simulink model "S250205simul_switch_2023a"  (R2024b)
settings: Solver=FixedStepDiscrete  StartTime=0  StopTime=60  FixedStep=0.01  RelTol=1e-3  AbsTol=1e-6
undefined symbols (not defined in the file or in its folder): a, b, c, d, f, g, switch_logic, VmcRgn_C_C, VmcRgn_J_C, VmcRgn_k_1to2_C, VmcRgn_k_2to3_C, VmcRgn_k_2to6_C, VmcRgn_k_3to4_C, VmcRgn_k_5to2_C, VmcRgn_k_6to2_C, VmcRgn_Kp_C, VmcRgn_L_C, VmcRgn_lf_C, VmcRgn_lr_C, VmcRgn_mass_C, VmcRgn_Mot2Whl_C, VmcRgn_PedDep_thrs_C, VmcRgn_phs2_k_C, VmcRgn_phs2_tq_C, VmcRgn_phs3_tq_C, VmcRgn_phs4_tq_C, VmcRgn_phs5_tq_C, VmcRgn_phs6_tq_C, VmcRgn_r_e_C, VmcRgn_R_whl_C, VmcRgn_SAS_thrs_C, VmcRgn_slip_max_C, VmcRgn_slip_max_gain_F_C, VmcRgn_slip_max_gain_R_C, VmcRgn_sup_tq_C, VmcRgn_t_pred_C, VmcRgn_target_w_acc_C, VmcRgn_tTs, VmcRgn_tTsinMs_C, VmcRgn_Yaw_thrs_C, yaw_flag
libraries: simulink x26, simulink_need_slupdate x1
(part 2 of 3)

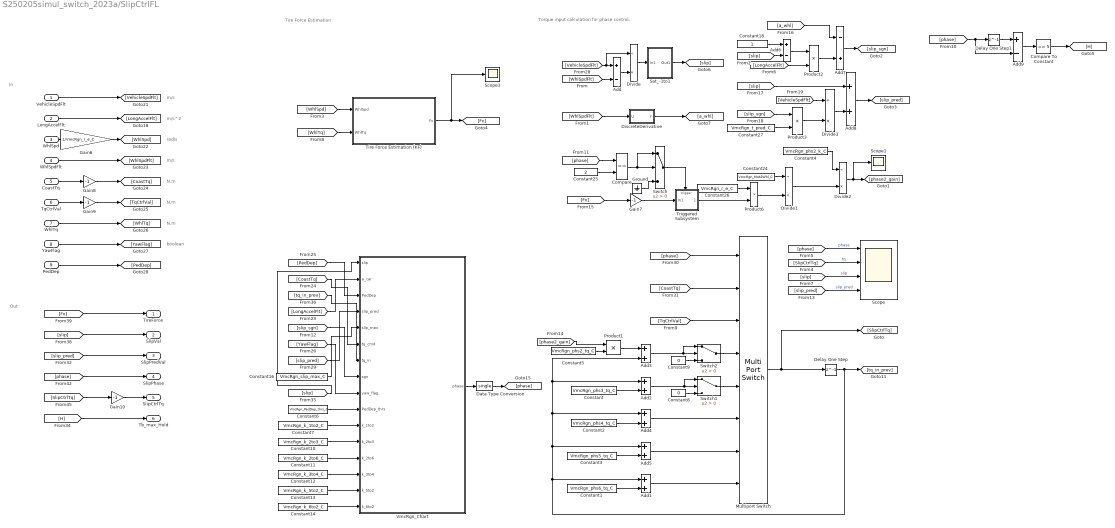
== system S250205simul_switch_2023a/SlipCtrlFL ==
  note: m/s
  note: N.m
  note: boolean
  note: N.m
  note: m/s
  note: Torque input calculation for phase control.
  note: Out
  note: N.m
  note: rad/s
  note: Tire Force Estimation
  note: m/s^2
  note: In
  VehicleSpdFlt : Inport
  LongAccelFlt : Inport  Port=2
  WhlSpd : Inport  Port=3
  WhlSpdFlt : Inport  Port=4
  CoastTq : Inport  Port=5
  TqCtrlVal : Inport  Port=6
  WhlTq : Inport  Port=7
  YawFlag : Inport  Port=8
  PedDep : Inport  Port=9
  Add : Sum  Inputs=+-
  Add{1..5,8} (6 alike) : Sum
  Add6 : Sum  Inputs=+-
  Add7 : Sum  Inputs=-+
  Add9 : Sum  Inputs=+-
  Compare : RelationalOperator  Operator===  OutDataTypeStr=boolean
  Compare To Constant : simulink/Logic and Bit Operations/Compare To Constant  relop===  const=5  OutDataTypeStr=boolean
  Constant : Constant  Value=VmcRgn_phs3_tq_C  OutDataTypeStr=single
  Constant1 : Constant  Value=VmcRgn_phs6_tq_C  OutDataTypeStr=single
  Constant10 : Constant  Value=VmcRgn_k_2to3_C  OutDataTypeStr=single
  Constant11 : Constant  Value=VmcRgn_k_2to6_C  OutDataTypeStr=single
  Constant12 : Constant  Value=VmcRgn_k_3to4_C  OutDataTypeStr=single
  Constant13 : Constant  Value=VmcRgn_k_5to2_C  OutDataTypeStr=single
  Constant14 : Constant  Value=VmcRgn_k_6to2_C  OutDataTypeStr=single
  Constant16 : Constant  Value=VmcRgn_slip_max_C  OutDataTypeStr=single
  Constant18 : Constant  OutDataTypeStr=single
  Constant2 : Constant  Value=VmcRgn_phs4_tq_C  OutDataTypeStr=single
  Constant24 : Constant  Value=VmcRgn_Mot2Whl_C  OutDataTypeStr=single
  Constant25 : Constant  Value=2  OutDataTypeStr=single
  Constant26 : Constant  Value=VmcRgn_r_e_C  OutDataTypeStr=single
  Constant27 : Constant  Value=VmcRgn_t_pred_C  OutDataTypeStr=single
  Constant3 : Constant  Value=VmcRgn_phs5_tq_C  OutDataTypeStr=single
  Constant4 : Constant  Value=VmcRgn_phs2_k_C  OutDataTypeStr=single
  Constant5 : Constant  Value=VmcRgn_phs2_tq_C  OutDataTypeStr=single
  Constant6 : Constant  Value=VmcRgn_PedDep_thrs_C  OutDataTypeStr=single
  Constant7 : Constant  Value=VmcRgn_k_1to2_C  OutDataTypeStr=single
  Constant8 : Constant  Value=0  OutDataTypeStr=single
  Constant9 : Constant  Value=0  OutDataTypeStr=single
  Data Type Conversion : DataTypeConversion  OutDataTypeStr=single  SaturateOnIntegerOverflow=off  RndMeth=Floor
  Delay One Step : Delay  DelayLength=1
  Delay One Step1 : Delay  DelayLength=1
  DiscreteDerivative : Subsystem  TreatAsAtomicUnit=on  RTWFileName=HmcLib_DebFlt  mask(Discrete Derivative with fixed sample time){Ts=VmcRgn_tTsinMs_C, out_type=single}
      mask prompts: Ts "Sampling Period [ms]"; out_type "Output DataType:"
      mask help:
      | Discrete-time derivative of the input.
      |
      | * Notes
      |   - Internal data type: Float32 (single)
      settings: AttributesFormatString=Sampling Period [ms]: %<Ts>\nOutType: %<out_type>  RTWSystemCode=Inline
  Divide : Product  Inputs=/*  OutDataTypeStr=single
  Divide1 : Product  Inputs=/*
  Divide2 : Product  Inputs=/*
  Divide3 : Product  Inputs=/*
  Gain{7..10} (4 alike) : Gain  Gain=-1
  Gain6 : Gain  Gain=1/VmcRgn_r_e_C
  Ground : Ground
  Multiport Switch : MultiPortSwitch  DataPortOrder=Zero-based contiguous  Inputs=7  zeroidx=on  OutDataTypeStr=single  SaturateOnIntegerOverflow=off  InputSameDT=off
  Product{1..3,6} (4 alike) : Product
  Sat_-1to1 : Subsystem
  Scope : Scope  NumInputPorts=4
  Scope1 : Scope
  Scope3 : Scope
  Switch : Switch  Criteria=u2 > Threshold  SaturateOnIntegerOverflow=off  InputSameDT=off
  Switch1 : Switch  Criteria=u2 > Threshold  SaturateOnIntegerOverflow=off  InputSameDT=off
  Switch2 : Switch  Criteria=u2 > Threshold  SaturateOnIntegerOverflow=off  InputSameDT=off
  Tire Force Estimation (KF) : Subsystem
  Triggered Subsystem : Subsystem  TreatAsAtomicUnit=on
  VmcRgn_Chart : Stateflow chart  TreatAsAtomicUnit=on
  TireForce : Outport
  SlipVal : Outport  Port=2
  SlipPredVal : Outport  Port=3
  SlipPhase : Outport  Port=4
  SlipCtrlTq : Outport  Port=5
  Tb_max_Hold : Outport  Port=6
  wires:
  [WhlSpd] -> Tire Force Estimation (KF)/1(WhlSpd)
  Data Type Conversion/1 -> [phase]
  Product3/1 -> Divide3/2
  Product2/1 -> Add7/2
  VmcRgn_Chart/1(phase) -> Data Type Conversion/1
  Divide3/1 -> Add8/2
  [slip] -> Add8/1
  [LongAccelFlt] -> Product2/2
  Switch2/1 -> Multiport Switch/4
  Add8/1 -> [slip_pred]
  Constant9/1 -> Switch2/3
  Delay One Step/1 -> [tq_in_prev], Add1/1, Add3/2, Add2/1, Add4/1, Add5/1
  [slip_sgn] -> Product3/1
  Constant26/1 -> Product6/1
  Triggered Subsystem/1(Out1) -> Product6/2
  Divide1/1 -> Divide2/2
  Constant4/1 -> Divide2/1
  Switch/1 -> Triggered Subsystem/Trigger
  Constant24/1 -> Divide1/1
  Product6/1 -> Divide1/2
  Ground/1 -> Switch/3
  [VehicleSpdFlt] -> Divide/1, Add/1
  Sat_-1to1/1(Out1) -> [slip]
  [WhlSpdFlt] -> DiscreteDerivative/1(U)
  [slip] -> Add6/2
  Constant1/1 -> Add1/2
  [slip_pred] -> Scope/4  "slip_pred"
  Add3/1 -> Switch2/1, Switch2/2
  [WhlTq] -> Tire Force Estimation (KF)/2(WhlTq)
  Add2/1 -> Switch1/1, Switch1/2
  [LongAccelFlt] -> VmcRgn_Chart/2(a_car)
  [SlipCtrlTq] -> Scope/2  "tq"
  [tq_in_prev] -> VmcRgn_Chart/7(tq_in)
  [WhlSpdFlt] -> Add/2
  [phase] -> Scope/1  "phase"
  Add6/1 -> Product2/1
  Gain8/1 -> [CoastTq]
  WhlSpd/1 -> Gain6/1
  YawFlag/1 -> [YawFlag]
  Multiport Switch/1 -> [SlipCtrlTq], Delay One Step/1
  CoastTq/1 -> Gain8/1
  Add4/1 -> Multiport Switch/6
  Constant3/1 -> Add5/2
  Divide/1 -> Sat_-1to1/1(In1)
  Constant27/1 -> Product3/2
  [phase] -> Compare/1
  Constant2/1 -> Add4/2
  Constant6/1 -> VmcRgn_Chart/10(PedDep_thrs)
  [phase2_gain] -> Product1/1
  [slip_sgn] -> VmcRgn_Chart/8(sgn)
  [slip] -> Scope/3  "slip"
  Constant/1 -> Add2/2
  Add5/1 -> Multiport Switch/7
  Constant14/1 -> VmcRgn_Chart/16(k_6to2)
  [YawFlag] -> VmcRgn_Chart/9(yaw_flag)
  Constant8/1 -> Switch1/3
  Constant10/1 -> VmcRgn_Chart/12(k_2to3)
  Constant7/1 -> VmcRgn_Chart/11(k_1to2)
  [CoastTq] -> VmcRgn_Chart/6(tq_cmd)
  [slip_pred] -> VmcRgn_Chart/4(slip_pred)
  Constant13/1 -> VmcRgn_Chart/15(k_5to2)
  Constant25/1 -> Compare/2
  Constant18/1 -> Add6/1
  [slip_pred] -> SlipPredVal/1
  Tire Force Estimation (KF)/1(Fx) -> Scope3/1, [Fx]
  Divide2/1 -> Scope1/1, [phase2_gain]
  Product1/1 -> Add3/1
  Gain6/1 -> [WhlSpd]
  Gain10/1 -> SlipCtrlTq/1
  Constant11/1 -> VmcRgn_Chart/13(k_2to6)
  LongAccelFlt/1 -> [LongAccelFlt]
  Compare/1 -> Switch/1, Switch/2
  [CoastTq] -> Multiport Switch/2
  Add7/1 -> [slip_sgn]
  Gain9/1 -> [TqCtrlVal]
  DiscreteDerivative/1(Y) -> [a_whl]
  [Fx] -> TireForce/1
  [slip] -> SlipVal/1
  [phase] -> SlipPhase/1
  WhlSpdFlt/1 -> [WhlSpdFlt]
  [SlipCtrlTq] -> Gain10/1
  WhlTq/1 -> [WhlTq]
  [slip] -> VmcRgn_Chart/1(slip)
  TqCtrlVal/1 -> Gain9/1
  [phase] -> Multiport Switch/1
  PedDep/1 -> [PedDep]
  Gain7/1 -> Triggered Subsystem/1(In1)
  [PedDep] -> VmcRgn_Chart/3(PedDep)
  [TqCtrlVal] -> Multiport Switch/3
  Constant12/1 -> VmcRgn_Chart/14(k_3to4)
  Switch1/1 -> Multiport Switch/5
  Add/1 -> Divide/2
  Add1/1 -> Multiport Switch/8
  [VehicleSpdFlt] -> Divide3/1
  VehicleSpdFlt/1 -> [VehicleSpdFlt]
  [Fx] -> Gain7/1
  Constant16/1 -> VmcRgn_Chart/5(slip_max)
  Constant5/1 -> Product1/2
  [a_whl] -> Add7/1
  [phase] -> Add9/2, Delay One Step1/1
  Compare To Constant/1 -> [H]
  Add9/1 -> Compare To Constant/1
  Delay One Step1/1 -> Add9/1
  [H] -> Tb_max_Hold/1

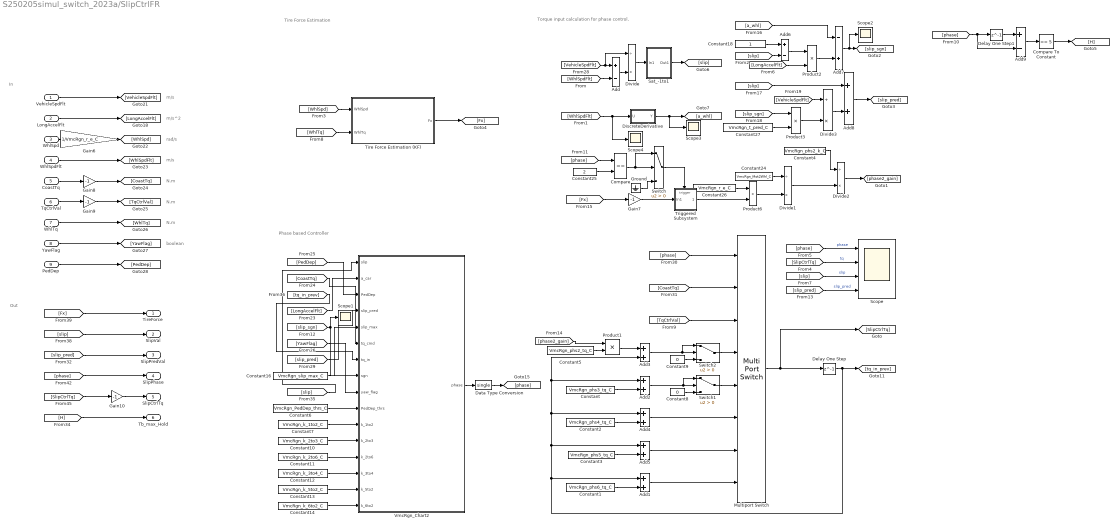
== system S250205simul_switch_2023a/SlipCtrlFR ==
  note: Phase based Controller
  note: m/s
  note: N.m
  note: boolean
  note: N.m
  note: m/s
  note: Torque input calculation for phase control.
  note: Out
  note: N.m
  note: rad/s
  note: Tire Force Estimation
  note: m/s^2
  note: In
  VehicleSpdFlt : Inport
  LongAccelFlt : Inport  Port=2
  WhlSpd : Inport  Port=3
  WhlSpdFlt : Inport  Port=4
  CoastTq : Inport  Port=5
  TqCtrlVal : Inport  Port=6
  WhlTq : Inport  Port=7
  YawFlag : Inport  Port=8
  PedDep : Inport  Port=9
  Add : Sum  Inputs=+-
  Add{1..5,8} (6 alike) : Sum
  Add6 : Sum  Inputs=+-
  Add7 : Sum  Inputs=-+
  Add9 : Sum  Inputs=+-
  Compare : RelationalOperator  Operator===  OutDataTypeStr=boolean
  Compare To Constant : simulink/Logic and Bit Operations/Compare To Constant  relop===  const=5  OutDataTypeStr=boolean
  Constant : Constant  Value=VmcRgn_phs3_tq_C  OutDataTypeStr=single
  Constant1 : Constant  Value=VmcRgn_phs6_tq_C  OutDataTypeStr=single
  Constant10 : Constant  Value=VmcRgn_k_2to3_C  OutDataTypeStr=single
  Constant11 : Constant  Value=VmcRgn_k_2to6_C  OutDataTypeStr=single
  Constant12 : Constant  Value=VmcRgn_k_3to4_C  OutDataTypeStr=single
  Constant13 : Constant  Value=VmcRgn_k_5to2_C  OutDataTypeStr=single
  Constant14 : Constant  Value=VmcRgn_k_6to2_C  OutDataTypeStr=single
  Constant16 : Constant  Value=VmcRgn_slip_max_C  OutDataTypeStr=single
  Constant18 : Constant  OutDataTypeStr=single
  Constant2 : Constant  Value=VmcRgn_phs4_tq_C  OutDataTypeStr=single
  Constant24 : Constant  Value=VmcRgn_Mot2Whl_C  OutDataTypeStr=single
  Constant25 : Constant  Value=2  OutDataTypeStr=single
  Constant26 : Constant  Value=VmcRgn_r_e_C  OutDataTypeStr=single
  Constant27 : Constant  Value=VmcRgn_t_pred_C  OutDataTypeStr=single
  Constant3 : Constant  Value=VmcRgn_phs5_tq_C  OutDataTypeStr=single
  Constant4 : Constant  Value=VmcRgn_phs2_k_C  OutDataTypeStr=single
  Constant5 : Constant  Value=VmcRgn_phs2_tq_C  OutDataTypeStr=single
  Constant6 : Constant  Value=VmcRgn_PedDep_thrs_C  OutDataTypeStr=single
  Constant7 : Constant  Value=VmcRgn_k_1to2_C  OutDataTypeStr=single
  Constant8 : Constant  Value=0  OutDataTypeStr=single
  Constant9 : Constant  Value=0  OutDataTypeStr=single
  Data Type Conversion : DataTypeConversion  OutDataTypeStr=single  SaturateOnIntegerOverflow=off  RndMeth=Floor
  Delay One Step : Delay  DelayLength=1
  Delay One Step1 : Delay  DelayLength=1
  DiscreteDerivative : Subsystem  TreatAsAtomicUnit=on  RTWFileName=HmcLib_DebFlt  mask(Discrete Derivative with fixed sample time){Ts=VmcRgn_tTsinMs_C, out_type=single}
      mask prompts: Ts "Sampling Period [ms]"; out_type "Output DataType:"
      mask help:
      | Discrete-time derivative of the input.
      |
      | * Notes
      |   - Internal data type: Float32 (single)
      settings: AttributesFormatString=Sampling Period [ms]: %<Ts>\nOutType: %<out_type>  RTWSystemCode=Inline
  Divide : Product  Inputs=/*  OutDataTypeStr=single
  Divide1 : Product  Inputs=/*
  Divide2 : Product  Inputs=/*
  Divide3 : Product  Inputs=/*
  Gain{7..10} (4 alike) : Gain  Gain=-1
  Gain6 : Gain  Gain=1/VmcRgn_r_e_C
  Ground : Ground
  Multiport Switch : MultiPortSwitch  DataPortOrder=Zero-based contiguous  Inputs=7  zeroidx=on  OutDataTypeStr=single  SaturateOnIntegerOverflow=off  InputSameDT=off
  Product{1..3,6} (4 alike) : Product
  Sat_-1to1 : Subsystem
  Scope : Scope  NumInputPorts=4
  Scope{1..4} (4 alike) : Scope
  Switch : Switch  Criteria=u2 > Threshold  SaturateOnIntegerOverflow=off  InputSameDT=off
  Switch1 : Switch  Criteria=u2 > Threshold  SaturateOnIntegerOverflow=off  InputSameDT=off
  Switch2 : Switch  Criteria=u2 > Threshold  SaturateOnIntegerOverflow=off  InputSameDT=off
  Tire Force Estimation (KF) : Subsystem
  Triggered Subsystem : Subsystem  TreatAsAtomicUnit=on
  VmcRgn_Chart2 : Stateflow chart  TreatAsAtomicUnit=on
  TireForce : Outport
  SlipVal : Outport  Port=2
  SlipPredVal : Outport  Port=3
  SlipPhase : Outport  Port=4
  SlipCtrlTq : Outport  Port=5
  Tb_max_Hold : Outport  Port=6
  wires:
  [WhlSpd] -> Tire Force Estimation (KF)/1(WhlSpd)
  Data Type Conversion/1 -> [phase]
  Product3/1 -> Divide3/2
  Product2/1 -> Add7/2
  VmcRgn_Chart2/1(phase) -> Data Type Conversion/1
  Divide3/1 -> Add8/2
  [slip] -> Add8/1
  [LongAccelFlt] -> Product2/2
  Switch2/1 -> Multiport Switch/4
  Add8/1 -> [slip_pred]
  Constant9/1 -> Switch2/3
  Delay One Step/1 -> [tq_in_prev], Add1/1, Add3/2, Add2/1, Add4/1, Add5/1
  [slip_sgn] -> Product3/1
  Constant26/1 -> Product6/1
  Triggered Subsystem/1(Out1) -> Product6/2
  Divide1/1 -> Divide2/2
  Constant4/1 -> Divide2/1
  Switch/1 -> Triggered Subsystem/Trigger
  Constant24/1 -> Divide1/1
  Product6/1 -> Divide1/2
  Ground/1 -> Switch/3
  [VehicleSpdFlt] -> Divide/1, Add/1
  Sat_-1to1/1(Out1) -> [slip]
  [WhlSpdFlt] -> DiscreteDerivative/1(U), Scope4/1
  [slip] -> Add6/2
  Constant1/1 -> Add1/2
  [slip_pred] -> Scope/4  "slip_pred"
  Add3/1 -> Switch2/1, Switch2/2
  [WhlTq] -> Tire Force Estimation (KF)/2(WhlTq)
  Add2/1 -> Switch1/1, Switch1/2
  [LongAccelFlt] -> VmcRgn_Chart2/2(a_car)
  [SlipCtrlTq] -> Scope/2  "tq"
  [tq_in_prev] -> VmcRgn_Chart2/7(tq_in)
  [WhlSpdFlt] -> Add/2
  [phase] -> Scope/1  "phase"
  Add6/1 -> Product2/1
  Gain8/1 -> [CoastTq]
  WhlSpd/1 -> Gain6/1
  YawFlag/1 -> [YawFlag]
  Multiport Switch/1 -> [SlipCtrlTq], Delay One Step/1
  CoastTq/1 -> Gain8/1
  Add4/1 -> Multiport Switch/6
  Constant3/1 -> Add5/2
  Divide/1 -> Sat_-1to1/1(In1)
  Constant27/1 -> Product3/2
  [phase] -> Compare/1
  Constant2/1 -> Add4/2
  Constant6/1 -> VmcRgn_Chart2/10(PedDep_thrs)
  [phase2_gain] -> Product1/1
  [slip_sgn] -> Scope1/1, VmcRgn_Chart2/8(sgn)
  [slip] -> Scope/3  "slip"
  Constant/1 -> Add2/2
  Add5/1 -> Multiport Switch/7
  Constant14/1 -> VmcRgn_Chart2/16(k_6to2)
  [YawFlag] -> VmcRgn_Chart2/9(yaw_flag)
  Constant8/1 -> Switch1/3
  Constant10/1 -> VmcRgn_Chart2/12(k_2to3)
  Constant7/1 -> VmcRgn_Chart2/11(k_1to2)
  [CoastTq] -> VmcRgn_Chart2/6(tq_cmd)
  [slip_pred] -> VmcRgn_Chart2/4(slip_pred)
  Constant13/1 -> VmcRgn_Chart2/15(k_5to2)
  Constant25/1 -> Compare/2
  Constant18/1 -> Add6/1
  [slip_pred] -> SlipPredVal/1
  Tire Force Estimation (KF)/1(Fx) -> [Fx]
  Divide2/1 -> [phase2_gain]
  Product1/1 -> Add3/1
  Gain6/1 -> [WhlSpd]
  Gain10/1 -> SlipCtrlTq/1
  Constant11/1 -> VmcRgn_Chart2/13(k_2to6)
  LongAccelFlt/1 -> [LongAccelFlt]
  Compare/1 -> Switch/1, Switch/2
  [CoastTq] -> Multiport Switch/2
  Add7/1 -> Scope2/1, [slip_sgn]
  Gain9/1 -> [TqCtrlVal]
  DiscreteDerivative/1(Y) -> Scope3/1, [a_whl]
  [Fx] -> TireForce/1
  [slip] -> SlipVal/1
  [phase] -> SlipPhase/1
  WhlSpdFlt/1 -> [WhlSpdFlt]
  [SlipCtrlTq] -> Gain10/1
  WhlTq/1 -> [WhlTq]
  [slip] -> VmcRgn_Chart2/1(slip)
  TqCtrlVal/1 -> Gain9/1
  [phase] -> Multiport Switch/1
  PedDep/1 -> [PedDep]
  Gain7/1 -> Triggered Subsystem/1(In1)
  [PedDep] -> VmcRgn_Chart2/3(PedDep)
  [TqCtrlVal] -> Multiport Switch/3
  Constant12/1 -> VmcRgn_Chart2/14(k_3to4)
  Switch1/1 -> Multiport Switch/5
  Add/1 -> Divide/2
  Add1/1 -> Multiport Switch/8
  [VehicleSpdFlt] -> Divide3/1
  VehicleSpdFlt/1 -> [VehicleSpdFlt]
  [Fx] -> Gain7/1
  Constant16/1 -> VmcRgn_Chart2/5(slip_max)
  Constant5/1 -> Product1/2
  [a_whl] -> Add7/1
  [phase] -> Add9/2, Delay One Step1/1
  Compare To Constant/1 -> [H]
  Add9/1 -> Compare To Constant/1
  Delay One Step1/1 -> Add9/1
  [H] -> Tb_max_Hold/1

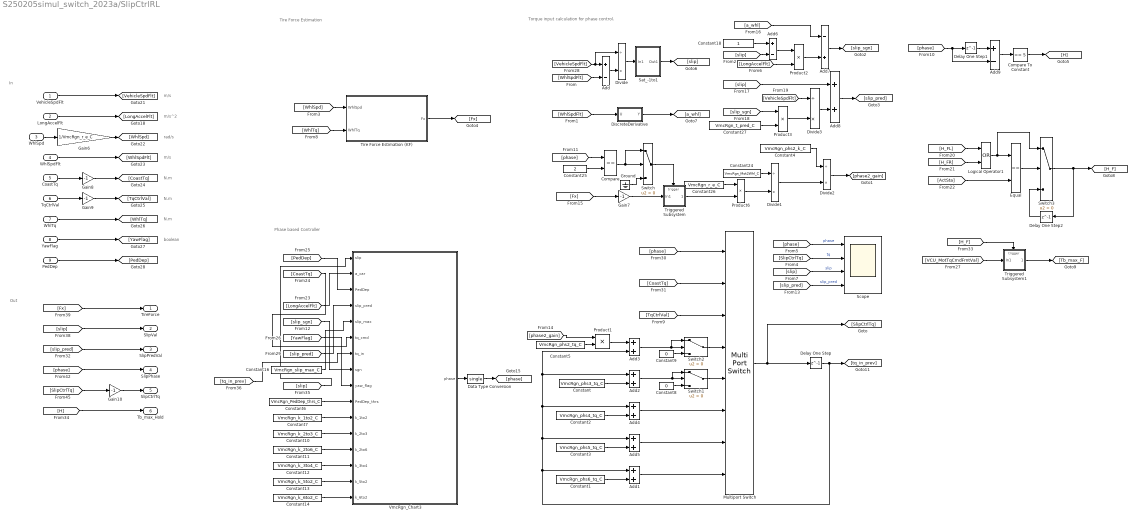
== system S250205simul_switch_2023a/SlipCtrlRL ==
  note: Phase based Controller
  note: m/s
  note: N.m
  note: boolean
  note: N.m
  note: m/s
  note: Torque input calculation for phase control.
  note: Out
  note: N.m
  note: rad/s
  note: Tire Force Estimation
  note: m/s^2
  note: In
  VehicleSpdFlt : Inport
  LongAccelFlt : Inport  Port=2
  WhlSpd : Inport  Port=3
  WhlSpdFlt : Inport  Port=4
  CoastTq : Inport  Port=5
  TqCtrlVal : Inport  Port=6
  WhlTq : Inport  Port=7
  YawFlag : Inport  Port=8
  PedDep : Inport  Port=9
  Add : Sum  Inputs=+-
  Add{1..5,8} (6 alike) : Sum
  Add6 : Sum  Inputs=+-
  Add7 : Sum  Inputs=-+
  Add9 : Sum  Inputs=+-
  Compare : RelationalOperator  Operator===  OutDataTypeStr=boolean
  Compare To Constant : simulink/Logic and Bit Operations/Compare To Constant  relop===  const=5  OutDataTypeStr=boolean
  Constant : Constant  Value=VmcRgn_phs3_tq_C  OutDataTypeStr=single
  Constant1 : Constant  Value=VmcRgn_phs6_tq_C  OutDataTypeStr=single
  Constant10 : Constant  Value=VmcRgn_k_2to3_C  OutDataTypeStr=single
  Constant11 : Constant  Value=VmcRgn_k_2to6_C  OutDataTypeStr=single
  Constant12 : Constant  Value=VmcRgn_k_3to4_C  OutDataTypeStr=single
  Constant13 : Constant  Value=VmcRgn_k_5to2_C  OutDataTypeStr=single
  Constant14 : Constant  Value=VmcRgn_k_6to2_C  OutDataTypeStr=single
  Constant16 : Constant  Value=VmcRgn_slip_max_C  OutDataTypeStr=single
  Constant18 : Constant  OutDataTypeStr=single
  Constant2 : Constant  Value=VmcRgn_phs4_tq_C  OutDataTypeStr=single
  Constant24 : Constant  Value=VmcRgn_Mot2Whl_C  OutDataTypeStr=single
  Constant25 : Constant  Value=2  OutDataTypeStr=single
  Constant26 : Constant  Value=VmcRgn_r_e_C  OutDataTypeStr=single
  Constant27 : Constant  Value=VmcRgn_t_pred_C  OutDataTypeStr=single
  Constant3 : Constant  Value=VmcRgn_phs5_tq_C  OutDataTypeStr=single
  Constant4 : Constant  Value=VmcRgn_phs2_k_C  OutDataTypeStr=single
  Constant5 : Constant  Value=VmcRgn_phs2_tq_C  OutDataTypeStr=single
  Constant6 : Constant  Value=VmcRgn_PedDep_thrs_C  OutDataTypeStr=single
  Constant7 : Constant  Value=VmcRgn_k_1to2_C  OutDataTypeStr=single
  Constant8 : Constant  Value=0  OutDataTypeStr=single
  Constant9 : Constant  Value=0  OutDataTypeStr=single
  Data Type Conversion : DataTypeConversion  OutDataTypeStr=single  SaturateOnIntegerOverflow=off  RndMeth=Floor
  Delay One Step : Delay  DelayLength=1
  Delay One Step1 : Delay  DelayLength=1
  Delay One Step2 : Delay  DelayLength=1
  DiscreteDerivative : Subsystem  TreatAsAtomicUnit=on  RTWFileName=HmcLib_DebFlt  mask(Discrete Derivative with fixed sample time){Ts=VmcRgn_tTsinMs_C, out_type=single}
      mask prompts: Ts "Sampling Period [ms]"; out_type "Output DataType:"
      mask help:
      | Discrete-time derivative of the input.
      |
      | * Notes
      |   - Internal data type: Float32 (single)
      settings: AttributesFormatString=Sampling Period [ms]: %<Ts>\nOutType: %<out_type>  RTWSystemCode=Inline
  Divide : Product  Inputs=/*  OutDataTypeStr=single
  Divide1 : Product  Inputs=/*
  Divide2 : Product  Inputs=/*
  Divide3 : Product  Inputs=/*
  Equal : RelationalOperator  Operator===  OutDataTypeStr=boolean  RndMeth=Simplest  InputSameDT=off
  Gain{7..10} (4 alike) : Gain  Gain=-1
  Gain6 : Gain  Gain=1/VmcRgn_r_e_C
  Ground : Ground
  Logical Operator1 : Logic  Operator=OR  AllPortsSameDT=off  OutDataTypeStr=boolean
  Multiport Switch : MultiPortSwitch  DataPortOrder=Zero-based contiguous  Inputs=7  zeroidx=on  OutDataTypeStr=single  SaturateOnIntegerOverflow=off  InputSameDT=off
  Product{1..3,6} (4 alike) : Product
  Sat_-1to1 : Subsystem
  Scope : Scope  NumInputPorts=4
  Switch{,1..3} (4 alike) : Switch  Criteria=u2 > Threshold  SaturateOnIntegerOverflow=off  InputSameDT=off
  Tire Force Estimation (KF) : Subsystem
  Triggered Subsystem : Subsystem  TreatAsAtomicUnit=on
  Triggered Subsystem1 : Subsystem  TreatAsAtomicUnit=on
  VmcRgn_Chart3 : Stateflow chart  TreatAsAtomicUnit=on
  TireForce : Outport
  SlipVal : Outport  Port=2
  SlipPredVal : Outport  Port=3
  SlipPhase : Outport  Port=4
  SlipCtrlTq : Outport  Port=5
  Tb_max_Hold : Outport  Port=6
  wires:
  [WhlSpd] -> Tire Force Estimation (KF)/1(WhlSpd)
  Data Type Conversion/1 -> [phase]
  Product3/1 -> Divide3/2
  Product2/1 -> Add7/2
  VmcRgn_Chart3/1(phase) -> Data Type Conversion/1
  Divide3/1 -> Add8/2
  [slip] -> Add8/1
  [LongAccelFlt] -> Product2/2
  Switch2/1 -> Multiport Switch/4
  Add8/1 -> [slip_pred]
  Constant9/1 -> Switch2/3
  Delay One Step/1 -> [tq_in_prev], Add1/1, Add3/2, Add2/1, Add4/1, Add5/1
  [slip_sgn] -> Product3/1
  Constant26/1 -> Product6/1
  Triggered Subsystem/1(Out1) -> Product6/2
  Divide1/1 -> Divide2/2
  Constant4/1 -> Divide2/1
  Switch/1 -> Triggered Subsystem/Trigger
  Constant24/1 -> Divide1/1
  Product6/1 -> Divide1/2
  Ground/1 -> Switch/3
  [VehicleSpdFlt] -> Divide/1, Add/1
  Sat_-1to1/1(Out1) -> [slip]
  [WhlSpdFlt] -> DiscreteDerivative/1(U)
  [slip] -> Add6/2
  Constant1/1 -> Add1/2
  [slip_pred] -> Scope/4  "slip_pred"
  Add3/1 -> Switch2/1, Switch2/2
  [WhlTq] -> Tire Force Estimation (KF)/2(WhlTq)
  Add2/1 -> Switch1/1, Switch1/2
  [LongAccelFlt] -> VmcRgn_Chart3/2(a_car)
  [SlipCtrlTq] -> Scope/2  "tq"
  [tq_in_prev] -> VmcRgn_Chart3/7(tq_in)
  [WhlSpdFlt] -> Add/2
  [phase] -> Scope/1  "phase"
  Add6/1 -> Product2/1
  Gain8/1 -> [CoastTq]
  WhlSpd/1 -> Gain6/1
  YawFlag/1 -> [YawFlag]
  Multiport Switch/1 -> [SlipCtrlTq], Delay One Step/1
  CoastTq/1 -> Gain8/1
  Add4/1 -> Multiport Switch/6
  Constant3/1 -> Add5/2
  Divide/1 -> Sat_-1to1/1(In1)
  Constant27/1 -> Product3/2
  [phase] -> Compare/1
  Constant2/1 -> Add4/2
  Constant6/1 -> VmcRgn_Chart3/10(PedDep_thrs)
  [phase2_gain] -> Product1/1
  [slip_sgn] -> VmcRgn_Chart3/8(sgn)
  [slip] -> Scope/3  "slip"
  Constant/1 -> Add2/2
  Add5/1 -> Multiport Switch/7
  Constant14/1 -> VmcRgn_Chart3/16(k_6to2)
  [YawFlag] -> VmcRgn_Chart3/9(yaw_flag)
  Constant8/1 -> Switch1/3
  Constant10/1 -> VmcRgn_Chart3/12(k_2to3)
  Constant7/1 -> VmcRgn_Chart3/11(k_1to2)
  [CoastTq] -> VmcRgn_Chart3/6(tq_cmd)
  [slip_pred] -> VmcRgn_Chart3/4(slip_pred)
  Constant13/1 -> VmcRgn_Chart3/15(k_5to2)
  Constant25/1 -> Compare/2
  Constant18/1 -> Add6/1
  [slip_pred] -> SlipPredVal/1
  Tire Force Estimation (KF)/1(Fx) -> [Fx]
  Divide2/1 -> [phase2_gain]
  Product1/1 -> Add3/1
  Gain6/1 -> [WhlSpd]
  Gain10/1 -> SlipCtrlTq/1
  Constant11/1 -> VmcRgn_Chart3/13(k_2to6)
  LongAccelFlt/1 -> [LongAccelFlt]
  Compare/1 -> Switch/1, Switch/2
  [CoastTq] -> Multiport Switch/2
  Add7/1 -> [slip_sgn]
  Gain9/1 -> [TqCtrlVal]
  DiscreteDerivative/1(Y) -> [a_whl]
  [Fx] -> TireForce/1
  [slip] -> SlipVal/1
  [phase] -> SlipPhase/1
  WhlSpdFlt/1 -> [WhlSpdFlt]
  [SlipCtrlTq] -> Gain10/1
  WhlTq/1 -> [WhlTq]
  [slip] -> VmcRgn_Chart3/1(slip)
  TqCtrlVal/1 -> Gain9/1
  [phase] -> Multiport Switch/1
  PedDep/1 -> [PedDep]
  Gain7/1 -> Triggered Subsystem/1(In1)
  [PedDep] -> VmcRgn_Chart3/3(PedDep)
  [TqCtrlVal] -> Multiport Switch/3
  Constant12/1 -> VmcRgn_Chart3/14(k_3to4)
  Switch1/1 -> Multiport Switch/5
  Add/1 -> Divide/2
  Add1/1 -> Multiport Switch/8
  [VehicleSpdFlt] -> Divide3/1
  VehicleSpdFlt/1 -> [VehicleSpdFlt]
  [Fx] -> Gain7/1
  Constant16/1 -> VmcRgn_Chart3/5(slip_max)
  Constant5/1 -> Product1/2
  [a_whl] -> Add7/1
  [phase] -> Add9/2, Delay One Step1/1
  Delay One Step1/1 -> Add9/1
  Add9/1 -> Compare To Constant/1
  Compare To Constant/1 -> [H]
  [H_FL] -> Logical Operator1/1
  [H_FR] -> Logical Operator1/2
  Logical Operator1/1 -> Switch3/1, Equal/1
  [ActSta] -> Equal/2
  Equal/1 -> Switch3/2
  Switch3/1 -> [H_F], Delay One Step2/1
  Delay One Step2/1 -> Switch3/3
  [VCU_MotTqCmdFrntVal] -> Triggered Subsystem1/1(In1)
  [H_F] -> Triggered Subsystem1/Trigger
  Triggered Subsystem1/1(Out1) -> [Tb_max_F]
  [H] -> Tb_max_Hold/1

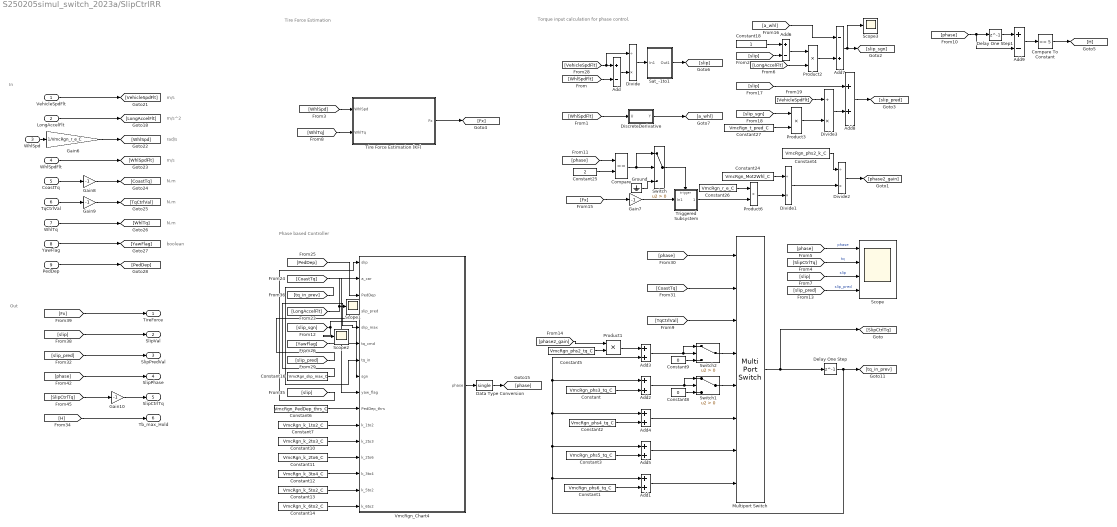
== system S250205simul_switch_2023a/SlipCtrlRR ==
  note: Phase based Controller
  note: m/s
  note: N.m
  note: boolean
  note: N.m
  note: m/s
  note: Torque input calculation for phase control.
  note: Out
  note: N.m
  note: rad/s
  note: Tire Force Estimation
  note: m/s^2
  note: In
  VehicleSpdFlt : Inport
  LongAccelFlt : Inport  Port=2
  WhlSpd : Inport  Port=3
  WhlSpdFlt : Inport  Port=4
  CoastTq : Inport  Port=5
  TqCtrlVal : Inport  Port=6
  WhlTq : Inport  Port=7
  YawFlag : Inport  Port=8
  PedDep : Inport  Port=9
  Add : Sum  Inputs=+-
  Add{1..5,8} (6 alike) : Sum
  Add6 : Sum  Inputs=+-
  Add7 : Sum  Inputs=-+
  Add9 : Sum  Inputs=+-
  Compare : RelationalOperator  Operator===  OutDataTypeStr=boolean
  Compare To Constant : simulink/Logic and Bit Operations/Compare To Constant  relop===  const=5  OutDataTypeStr=boolean
  Constant : Constant  Value=VmcRgn_phs3_tq_C  OutDataTypeStr=single
  Constant1 : Constant  Value=VmcRgn_phs6_tq_C  OutDataTypeStr=single
  Constant10 : Constant  Value=VmcRgn_k_2to3_C  OutDataTypeStr=single
  Constant11 : Constant  Value=VmcRgn_k_2to6_C  OutDataTypeStr=single
  Constant12 : Constant  Value=VmcRgn_k_3to4_C  OutDataTypeStr=single
  Constant13 : Constant  Value=VmcRgn_k_5to2_C  OutDataTypeStr=single
  Constant14 : Constant  Value=VmcRgn_k_6to2_C  OutDataTypeStr=single
  Constant16 : Constant  Value=VmcRgn_slip_max_C  OutDataTypeStr=single
  Constant18 : Constant  OutDataTypeStr=single
  Constant2 : Constant  Value=VmcRgn_phs4_tq_C  OutDataTypeStr=single
  Constant24 : Constant  Value=VmcRgn_Mot2Whl_C  OutDataTypeStr=single
  Constant25 : Constant  Value=2  OutDataTypeStr=single
  Constant26 : Constant  Value=VmcRgn_r_e_C  OutDataTypeStr=single
  Constant27 : Constant  Value=VmcRgn_t_pred_C  OutDataTypeStr=single
  Constant3 : Constant  Value=VmcRgn_phs5_tq_C  OutDataTypeStr=single
  Constant4 : Constant  Value=VmcRgn_phs2_k_C  OutDataTypeStr=single
  Constant5 : Constant  Value=VmcRgn_phs2_tq_C  OutDataTypeStr=single
  Constant6 : Constant  Value=VmcRgn_PedDep_thrs_C  OutDataTypeStr=single
  Constant7 : Constant  Value=VmcRgn_k_1to2_C  OutDataTypeStr=single
  Constant8 : Constant  Value=0  OutDataTypeStr=single
  Constant9 : Constant  Value=0  OutDataTypeStr=single
  Data Type Conversion : DataTypeConversion  OutDataTypeStr=single  SaturateOnIntegerOverflow=off  RndMeth=Floor
  Delay One Step : Delay  DelayLength=1
  Delay One Step1 : Delay  DelayLength=1
  DiscreteDerivative : Subsystem  TreatAsAtomicUnit=on  RTWFileName=HmcLib_DebFlt  mask(Discrete Derivative with fixed sample time){Ts=VmcRgn_tTsinMs_C, out_type=single}
      mask prompts: Ts "Sampling Period [ms]"; out_type "Output DataType:"
      mask help:
      | Discrete-time derivative of the input.
      |
      | * Notes
      |   - Internal data type: Float32 (single)
      settings: AttributesFormatString=Sampling Period [ms]: %<Ts>\nOutType: %<out_type>  RTWSystemCode=Inline
  Divide : Product  Inputs=/*  OutDataTypeStr=single
  Divide1 : Product  Inputs=/*
  Divide2 : Product  Inputs=/*
  Divide3 : Product  Inputs=/*
  Gain{7..10} (4 alike) : Gain  Gain=-1
  Gain6 : Gain  Gain=1/VmcRgn_r_e_C
  Ground : Ground
  Multiport Switch : MultiPortSwitch  DataPortOrder=Zero-based contiguous  Inputs=7  zeroidx=on  OutDataTypeStr=single  SaturateOnIntegerOverflow=off  InputSameDT=off
  Product{1..3,6} (4 alike) : Product
  Sat_-1to1 : Subsystem
  Scope : Scope  NumInputPorts=4
  Scope1 : Scope
  Scope2 : Scope
  Scope3 : Scope
  Switch : Switch  Criteria=u2 > Threshold  SaturateOnIntegerOverflow=off  InputSameDT=off
  Switch1 : Switch  Criteria=u2 > Threshold  SaturateOnIntegerOverflow=off  InputSameDT=off
  Switch2 : Switch  Criteria=u2 > Threshold  SaturateOnIntegerOverflow=off  InputSameDT=off
  Tire Force Estimation (KF) : Subsystem
  Triggered Subsystem : Subsystem  TreatAsAtomicUnit=on
  VmcRgn_Chart4 : Stateflow chart  TreatAsAtomicUnit=on
  TireForce : Outport
  SlipVal : Outport  Port=2
  SlipPredVal : Outport  Port=3
  SlipPhase : Outport  Port=4
  SlipCtrlTq : Outport  Port=5
  Tb_max_Hold : Outport  Port=6
  wires:
  [WhlSpd] -> Tire Force Estimation (KF)/1(WhlSpd)
  Data Type Conversion/1 -> [phase]
  Product3/1 -> Divide3/2
  Product2/1 -> Add7/2
  VmcRgn_Chart4/1(phase) -> Data Type Conversion/1
  Divide3/1 -> Add8/2
  [slip] -> Add8/1
  [LongAccelFlt] -> Product2/2
  Switch2/1 -> Multiport Switch/4
  Add8/1 -> [slip_pred]
  Constant9/1 -> Switch2/3
  Delay One Step/1 -> [tq_in_prev], Add1/1, Add3/2, Add2/1, Add4/1, Add5/1
  [slip_sgn] -> Product3/1
  Constant26/1 -> Product6/1
  Triggered Subsystem/1(Out1) -> Product6/2
  Divide1/1 -> Divide2/2
  Constant4/1 -> Divide2/1
  Switch/1 -> Triggered Subsystem/Trigger
  Constant24/1 -> Divide1/1
  Product6/1 -> Divide1/2
  Ground/1 -> Switch/3
  [VehicleSpdFlt] -> Divide/1, Add/1
  Sat_-1to1/1(Out1) -> [slip]
  [WhlSpdFlt] -> DiscreteDerivative/1(U)
  [slip] -> Add6/2
  Constant1/1 -> Add1/2
  [slip_pred] -> Scope/4  "slip_pred"
  Add3/1 -> Switch2/1, Switch2/2
  [WhlTq] -> Tire Force Estimation (KF)/2(WhlTq)
  Add2/1 -> Switch1/1, Switch1/2
  [LongAccelFlt] -> Scope1/1, VmcRgn_Chart4/2(a_car)
  [SlipCtrlTq] -> Scope/2  "tq"
  [tq_in_prev] -> VmcRgn_Chart4/7(tq_in)
  [WhlSpdFlt] -> Add/2
  [phase] -> Scope/1  "phase"
  Add6/1 -> Product2/1
  Gain8/1 -> [CoastTq]
  WhlSpd/1 -> Gain6/1
  YawFlag/1 -> [YawFlag]
  Multiport Switch/1 -> [SlipCtrlTq], Delay One Step/1
  CoastTq/1 -> Gain8/1
  Add4/1 -> Multiport Switch/6
  Constant3/1 -> Add5/2
  Divide/1 -> Sat_-1to1/1(In1)
  Constant27/1 -> Product3/2
  [phase] -> Compare/1
  Constant2/1 -> Add4/2
  Constant6/1 -> VmcRgn_Chart4/10(PedDep_thrs)
  [phase2_gain] -> Product1/1
  [slip_sgn] -> Scope2/1, VmcRgn_Chart4/8(sgn)
  [slip] -> Scope/3  "slip"
  Constant/1 -> Add2/2
  Add5/1 -> Multiport Switch/7
  Constant14/1 -> VmcRgn_Chart4/16(k_6to2)
  [YawFlag] -> VmcRgn_Chart4/9(yaw_flag)
  Constant8/1 -> Switch1/3
  Constant10/1 -> VmcRgn_Chart4/12(k_2to3)
  Constant7/1 -> VmcRgn_Chart4/11(k_1to2)
  [CoastTq] -> VmcRgn_Chart4/6(tq_cmd)
  [slip_pred] -> VmcRgn_Chart4/4(slip_pred)
  Constant13/1 -> VmcRgn_Chart4/15(k_5to2)
  Constant25/1 -> Compare/2
  Constant18/1 -> Add6/1
  [slip_pred] -> SlipPredVal/1
  Tire Force Estimation (KF)/1(Fx) -> [Fx]
  Divide2/1 -> [phase2_gain]
  Product1/1 -> Add3/1
  Gain6/1 -> [WhlSpd]
  Gain10/1 -> SlipCtrlTq/1
  Constant11/1 -> VmcRgn_Chart4/13(k_2to6)
  LongAccelFlt/1 -> [LongAccelFlt]
  Compare/1 -> Switch/1, Switch/2
  [CoastTq] -> Multiport Switch/2
  Add7/1 -> Scope3/1, [slip_sgn]
  Gain9/1 -> [TqCtrlVal]
  DiscreteDerivative/1(Y) -> [a_whl]
  [Fx] -> TireForce/1
  [slip] -> SlipVal/1
  [phase] -> SlipPhase/1
  WhlSpdFlt/1 -> [WhlSpdFlt]
  [SlipCtrlTq] -> Gain10/1
  WhlTq/1 -> [WhlTq]
  [slip] -> VmcRgn_Chart4/1(slip)
  TqCtrlVal/1 -> Gain9/1
  [phase] -> Multiport Switch/1
  PedDep/1 -> [PedDep]
  Gain7/1 -> Triggered Subsystem/1(In1)
  [PedDep] -> VmcRgn_Chart4/3(PedDep)
  [TqCtrlVal] -> Multiport Switch/3
  Constant12/1 -> VmcRgn_Chart4/14(k_3to4)
  Switch1/1 -> Multiport Switch/5
  Add/1 -> Divide/2
  Add1/1 -> Multiport Switch/8
  [VehicleSpdFlt] -> Divide3/1
  VehicleSpdFlt/1 -> [VehicleSpdFlt]
  [Fx] -> Gain7/1
  Constant16/1 -> VmcRgn_Chart4/5(slip_max)
  Constant5/1 -> Product1/2
  [a_whl] -> Add7/1
  [H] -> Tb_max_Hold/1
  [phase] -> Add9/2, Delay One Step1/1
  Compare To Constant/1 -> [H]
  Add9/1 -> Compare To Constant/1
  Delay One Step1/1 -> Add9/1

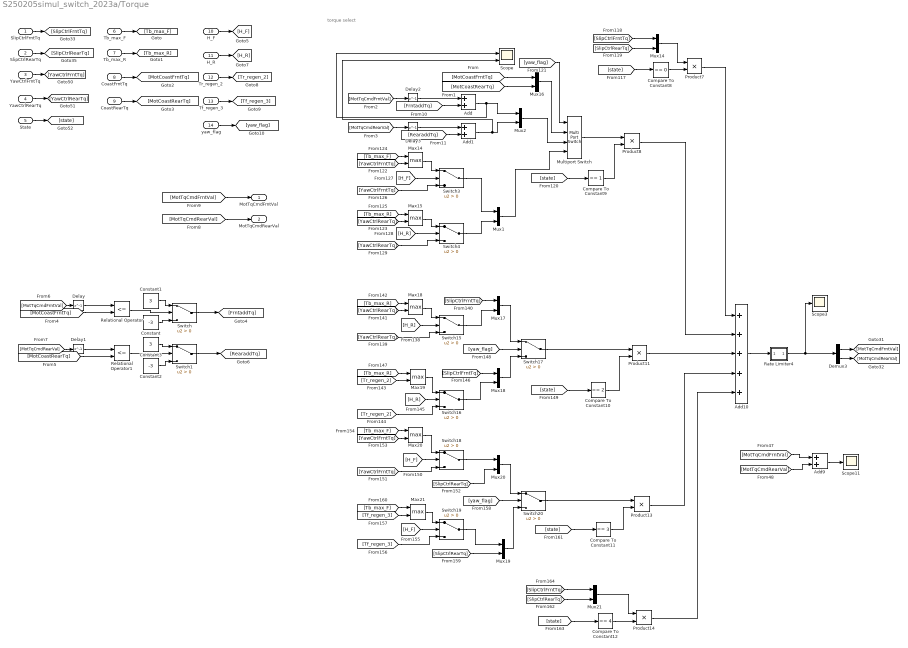
== system S250205simul_switch_2023a/Torque ==
  note: torque select
  SlipCtrlFrntTq : Inport
  SlipCtrlRearTq : Inport  Port=2
  YawCtrlFrntTq : Inport  Port=3
  YawCtrlRearTq : Inport  Port=4
  State : Inport  Port=5
  Tb_max_F : Inport  Port=6
  Tb_max_R : Inport  Port=7
  CoastFrntTq : Inport  Port=8
  CoastRearTq : Inport  Port=9
  H_F : Inport  Port=10
  H_R : Inport  Port=11
  Tr_regen_2 : Inport  Port=12
  Tf_regen_3 : Inport  Port=13
  yaw_flag : Inport  Port=14
  Add : Sum
  Add1 : Sum
  Add10 : Sum  Inputs=+++++  OutDataTypeStr=single
  Add9 : Sum  OutDataTypeStr=single
  Compare To Constant10 : simulink/Logic and Bit Operations/Compare To Constant  relop===  const=2  OutDataTypeStr=boolean
  Compare To Constant11 : simulink/Logic and Bit Operations/Compare To Constant  relop===  const=3  OutDataTypeStr=boolean
  Compare To Constant12 : simulink/Logic and Bit Operations/Compare To Constant  relop===  const=4  OutDataTypeStr=boolean
  Compare To Constant8 : simulink/Logic and Bit Operations/Compare To Constant  relop===  const=0  OutDataTypeStr=boolean
  Compare To Constant9 : simulink/Logic and Bit Operations/Compare To Constant  relop===  const=1  OutDataTypeStr=boolean
  Constant : Constant  Value=-3
  Constant1 : Constant  Value=3
  Constant2 : Constant  Value=-3
  Constant3 : Constant  Value=3
  Delay{,1..3} (4 alike) : Delay  DelayLength=1
  Demux3 : Demux  Outputs=2
  Max{14..15,18..21} (6 alike) : MinMax  Function=max  Inputs=2  OutDataTypeStr=single
  Multiport Switch : MultiPortSwitch  DataPortOrder=Zero-based contiguous  zeroidx=on  SaturateOnIntegerOverflow=off  InputSameDT=off
  Mux{1..2,14,16..21} (9 alike) : Mux  Inputs=2
  Product{7..8,11,13..14} (5 alike) : Product  OutDataTypeStr=single
  Rate Limiter4 : Subsystem
  Relational Operator : RelationalOperator  Operator=<=  OutDataTypeStr=boolean  RndMeth=Simplest  InputSameDT=off
  Relational Operator1 : RelationalOperator  Operator=<=  OutDataTypeStr=boolean  RndMeth=Simplest  InputSameDT=off
  Scope : Scope  NumInputPorts=2
  Scope11 : Scope
  Scope3 : Scope
  Switch : Switch  Criteria=u2 > Threshold  SaturateOnIntegerOverflow=off  InputSameDT=off
  Switch1 : Switch  Criteria=u2 > Threshold  SaturateOnIntegerOverflow=off  InputSameDT=off
  Switch{3..4,15..20} (8 alike) : Switch  Criteria=u2 > Threshold  OutDataTypeStr=single  SaturateOnIntegerOverflow=off  InputSameDT=off
  MotTqCmdFrntVal : Outport
  MotTqCmdRearVal : Outport  Port=2
  wires:
  [MotTqCmdFrntVal] -> Add9/1
  [MotTqCmdRearVal] -> Add9/2
  Add9/1 -> Scope11/1
  [state] -> Compare To Constant8/1
  Compare To Constant8/1 -> Product7/2
  [SlipCtrlFrntTq] -> Mux14/1
  [SlipCtrlRearTq] -> Mux14/2
  Mux14/1 -> Product7/1
  [state] -> Compare To Constant9/1
  Multiport Switch/1 -> Product8/1
  Compare To Constant9/1 -> Product8/2
  [Tb_max_R] -> Max18/1
  [YawCtrlRearTq] -> Switch15/3
  [H_R] -> Switch15/2
  [YawCtrlRearTq] -> Max18/2
  Max18/1 -> Switch15/1
  Max19/1 -> Switch16/1
  [H_R] -> Switch16/2
  [Tr_regen_2] -> Max19/2
  [Tb_max_R] -> Max19/1
  [SlipCtrlFrntTq] -> Mux17/1
  Switch15/1 -> Mux17/2
  [SlipCtrlFrntTq] -> Mux18/1
  Switch16/1 -> Mux18/2
  [Tr_regen_2] -> Switch16/3
  [yaw_flag] -> Switch17/2
  Mux17/1 -> Switch17/1
  Mux18/1 -> Switch17/3
  Switch17/1 -> Product11/1
  Compare To Constant10/1 -> Product11/2
  [state] -> Compare To Constant10/1
  [YawCtrlFrntTq] -> Switch18/3
  Max20/1 -> Switch18/1
  [YawCtrlFrntTq] -> Max20/2
  [Tb_max_F] -> Max20/1
  [H_F] -> Switch18/2
  Switch19/1 -> Mux19/1
  [H_F] -> Switch19/2
  [Tf_regen_3] -> Switch19/3
  Max21/1 -> Switch19/1
  [Tf_regen_3] -> Max21/2
  [SlipCtrlRearTq] -> Mux19/2
  [Tb_max_F] -> Max21/1
  Switch18/1 -> Mux20/1
  [SlipCtrlRearTq] -> Mux20/2
  [yaw_flag] -> Switch20/2
  Mux20/1 -> Switch20/1
  Mux19/1 -> Switch20/3
  [state] -> Compare To Constant11/1
  Switch20/1 -> Product13/1
  Compare To Constant11/1 -> Product13/2
  [state] -> Compare To Constant12/1
  [SlipCtrlRearTq] -> Mux21/2
  [SlipCtrlFrntTq] -> Mux21/1
  Compare To Constant12/1 -> Product14/2
  Mux21/1 -> Product14/1
  Product7/1 -> Add10/1
  Product8/1 -> Add10/2
  Product11/1 -> Add10/3
  Product13/1 -> Add10/4
  Product14/1 -> Add10/5
  Rate Limiter4/1(Out) -> Scope3/1, Demux3/1
  Demux3/2 -> [MotTqCmdRearVal]
  Demux3/1 -> [MotTqCmdFrntVal]
  Add10/1 -> Rate Limiter4/1(In)
  SlipCtrlFrntTq/1 -> [SlipCtrlFrntTq]
  SlipCtrlRearTq/1 -> [SlipCtrlRearTq]
  YawCtrlFrntTq/1 -> [YawCtrlFrntTq]
  YawCtrlRearTq/1 -> [YawCtrlRearTq]
  State/1 -> [state]
  [MotTqCmdFrntVal] -> MotTqCmdFrntVal/1
  [MotTqCmdRearVal] -> MotTqCmdRearVal/1
  Tb_max_F/1 -> [Tb_max_F]
  Tb_max_R/1 -> [Tb_max_R]
  CoastFrntTq/1 -> [MotCoastFrntTq]
  CoastRearTq/1 -> [MotCoastRearTq]
  H_F/1 -> [H_F]
  H_R/1 -> [H_R]
  Tr_regen_2/1 -> [Tr_regen_2]
  Tf_regen_3/1 -> [Tf_regen_3]
  yaw_flag/1 -> [yaw_flag]
  [MotCoastFrntTq] -> Mux16/1
  [MotCoastRearTq] -> Mux16/2
  [H_R] -> Switch4/2
  Max15/1 -> Switch4/1
  [Tb_max_F] -> Max14/1
  [YawCtrlFrntTq] -> Switch3/3
  [YawCtrlFrntTq] -> Max14/2
  [YawCtrlRearTq] -> Max15/2
  [Tb_max_R] -> Max15/1
  [YawCtrlRearTq] -> Switch4/3
  Max14/1 -> Switch3/1
  [H_F] -> Switch3/2
  [yaw_flag] -> Multiport Switch/1
  Mux1/1 -> Multiport Switch/4
  Switch3/1 -> Mux1/1
  Switch4/1 -> Mux1/2
  Mux16/1 -> Multiport Switch/2
  Mux2/1 -> Multiport Switch/3
  [MotTqCmdFrntVal] -> Delay/1
  [MotTqCmdRearVal] -> Delay1/1
  Delay/1 -> Relational Operator/1
  [MotCoastFrntTq] -> Relational Operator/2
  Delay1/1 -> Relational Operator1/1
  Relational Operator/1 -> Switch/2
  Constant/1 -> Switch/3
  Constant1/1 -> Switch/1
  Constant2/1 -> Switch1/3
  Constant3/1 -> Switch1/1
  Relational Operator1/1 -> Switch1/2
  Switch/1 -> [FrntaddTq]
  Switch1/1 -> [RearaddTq]
  [MotCoastRearTq] -> Relational Operator1/2
  [MotTqCmdFrntVal] -> Delay2/1
  [FrntaddTq] -> Add/2
  [MotTqCmdRearVal] -> Delay3/1
  [RearaddTq] -> Add1/2
  Add/1 -> Scope/1, Mux2/1
  Add1/1 -> Scope/2, Mux2/2
  Delay2/1 -> Add/1
  Delay3/1 -> Add1/1

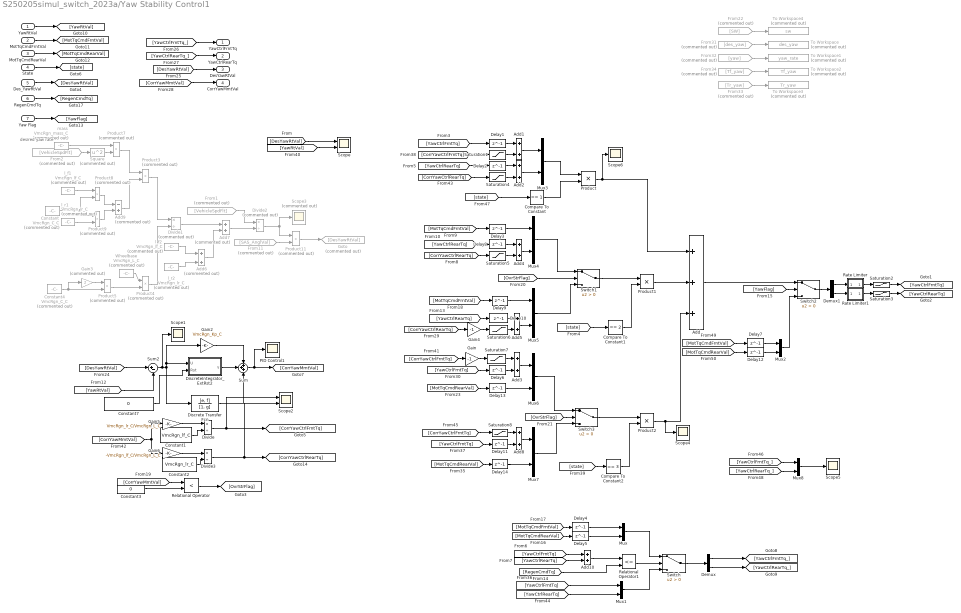
== system S250205simul_switch_2023a/Yaw Stability Control1 ==
  note: desired yaw rate
  YawRtVal : Inport  OutDataTypeStr=single
  MotTqCmdFrntVal : Inport  Port=2  OutDataTypeStr=single
  MotTqCmdRearVal : Inport  Port=3  OutDataTypeStr=single
  State : Inport  Port=4  OutDataTypeStr=single
  Des_YawRtVal : Inport  Port=5
  RegenCmdTq : Inport  Port=6
  Yaw Flag : Inport  Port=7
  Add : Sum  Inputs=+++
  Add{1..5,8,10} (7 alike) : Sum
  Add6 : Sum  Commented=on
  Add7 : Sum  Commented=on
  Add9 : Sum  Commented=on  Inputs=-+
  Compare To Constant : simulink/Logic and Bit Operations/Compare To Constant  relop===  const=1  OutDataTypeStr=boolean
  Compare To Constant1 : simulink/Logic and Bit Operations/Compare To Constant  relop===  const=2  OutDataTypeStr=boolean
  Compare To Constant2 : simulink/Logic and Bit Operations/Compare To Constant  relop===  const=3  OutDataTypeStr=boolean
  Constant : Constant  Commented=on  Value=VmcRgn_C_C  OutDataTypeStr=single
  Constant1 : Constant  Value=VmcRgn_lf_C  OutDataTypeStr=single
  Constant2 : Constant  Value=VmcRgn_lr_C  OutDataTypeStr=single
  Constant3 : Constant  Value=0
  Constant4 : Constant  Commented=on  Value=VmcRgn_C_C  OutDataTypeStr=single
  Constant7 : Constant  Value=0  OutDataTypeStr=boolean  LockScale=on  mask(Customized constant block){}
      settings: AttributesFormatString=OutType: %<OutDataTypeStr>
  Delay{1..14} (14 alike) : Delay  DelayLength=1
  Demux : Demux  Outputs=2
  Demux1 : Demux  Outputs=2
  Discrete Transfer Fcn : DiscreteTransferFcn  Numerator=[e, f]  Denominator=[1, g]
  DiscreteIntegrator_ExtRst2 : Subsystem  TreatAsAtomicUnit=on  RTWFileName=HmcLib_DebFlt  mask(Discrete Integrator with external reset){Ts=VmcRgn_tTsinMs_C, out_type=single}
      mask prompts: Ts "Sampling Period [ms]"; out_type "Output DataType:"
      mask help:
      | This block is a discrete integrator with external reset condition.
      |   - Inport1: Input value
      |   - Inport2: Reset signal (Boolean), Level detect
      |   - Outport1: Integrator value
      |
      | if R == False,
      |   Y[k] = Y[k-1] + Ts * U[k]
      | else, Y[K] = 0
      |
      | * Notes
      |   - Internal data type: Float32 (single)
      settings: AttributesFormatString=Sampling Period [ms]: %<Ts>\nOutType: %<out_type>  RTWSystemCode=Inline
      mask Display:
      | port_label('input', 1, 'U')
      | port_label('input', 2, 'RstRq_Bool')
      | port_label('output', 1, 'Y')
  Divide : Product  Inputs=*/
  Divide1 : Product  Commented=on  Inputs=*/
  Divide2 : Product  Commented=on  Inputs=*/
  Divide3 : Product  Inputs=*/
  From1 : From  Commented=on  GotoTag=VehicleSpdFlt
  From11 : From  Commented=on  GotoTag=SAS_AnglVal
  From2 : From  Commented=on  GotoTag=VehicleSpdFlt
  From22 : From  Commented=on  GotoTag=SW  TagVisibility=global
  From31 : From  Commented=on  GotoTag=des_yaw
  From32 : From  Commented=on  GotoTag=yaw  TagVisibility=global
  From33 : From  Commented=on  GotoTag=Tr_yaw
  From34 : From  Commented=on  GotoTag=Tf_yaw
  Gain : Gain  Gain=-1
  Gain2 : Gain  Gain=VmcRgn_Kp_C
  Gain3 : Gain  Commented=on  Gain=2  OutDataTypeStr=uint16
  Gain4 : Gain  Gain=-1
  Gain5 : Gain  Gain=VmcRgn_lr_C/VmcRgn_L_C
  Gain6 : Gain  Gain=-VmcRgn_lf_C/VmcRgn_L_C
  Goto : Goto  Commented=on  GotoTag=DesYawRtVal
  Mux{,1..8} (9 alike) : Mux  Inputs=2
  PID Control1 : Scope
  Product : Product  OutDataTypeStr=single
  Product1 : Product
  Product{3..5,7..9,11} (7 alike) : Product  Commented=on
  Product2 : Product
  Rate Limiter : Subsystem
  Rate Limiter1 : Subsystem
  Relational Operator : RelationalOperator  Operator=<  OutDataTypeStr=boolean  RndMeth=Simplest  InputSameDT=off
  Relational Operator1 : RelationalOperator  Operator=<=  OutDataTypeStr=boolean  RndMeth=Simplest  InputSameDT=off
  Saturation{1,4..8} (6 alike) : Saturate  UpperLimit=10  LowerLimit=-10
  Saturation2 : Saturate  UpperLimit=0  LowerLimit=-1000
  Saturation3 : Saturate  UpperLimit=0  LowerLimit=-1000
  Scope : Scope  NumInputPorts=2
  Scope{1,4..6} (4 alike) : Scope
  Scope2 : Scope  NumInputPorts=2
  Scope3 : Scope  Commented=on
  Square : Math  Commented=on  Operator=square  SignedPower=on
  Sum : Sum  Inputs=+++
  Sum2 : Sum  Inputs=|+-
  Switch{,1..3} (4 alike) : Switch  Criteria=u2 > Threshold  SaturateOnIntegerOverflow=off  InputSameDT=off
  To Workspace : ToWorkspace  Commented=on  VariableName=des_yaw  SaveFormat=Structure With Time  SampleTime=-1
  To Workspace1 : ToWorkspace  Commented=on  VariableName=yaw_rate  SaveFormat=Structure With Time  SampleTime=-1
  To Workspace2 : ToWorkspace  Commented=on  VariableName=Tf_yaw  SaveFormat=Structure With Time  SampleTime=-1
  To Workspace3 : ToWorkspace  Commented=on  VariableName=Tr_yaw  SaveFormat=Structure With Time  SampleTime=-1
  To Workspace4 : ToWorkspace  Commented=on  VariableName=sw  SaveFormat=Structure With Time  SampleTime=-1
  Wheelbase : Constant  Commented=on  Value=VmcRgn_L_C  OutDataTypeStr=single
  l_f1 : Constant  Commented=on  Value=VmcRgn_lf_C  OutDataTypeStr=single
  l_f2 : Constant  Commented=on  Value=VmcRgn_lf_C  OutDataTypeStr=single
  l_r1 : Constant  Commented=on  Value=VmcRgn_lr_C  OutDataTypeStr=single
  l_r2 : Constant  Commented=on  Value=VmcRgn_lr_C  OutDataTypeStr=single
  mass : Constant  Commented=on  Value=VmcRgn_mass_C  OutDataTypeStr=single
  YawCtrlFrntTq : Outport
  YawCtrlRearTq : Outport  Port=2
  DesYawRtVal : Outport  Port=3
  CorrYawMmtVal : Outport  Port=4
  wires:
  Constant7/1 -> DiscreteIntegrator_ExtRst2/2(Rst)
  Add9/1 -> Product3/2
  Add6/1 -> Add7/2
  l_r2/1 -> Add6/2
  Square/1 -> Product7/2
  l_f2/1 -> Add6/1
  Product4/1 -> Divide1/2
  Product7/1 -> Product3/1
  Gain3/1 -> Product5/1
  Product5/1 -> Product4/2
  Divide2/1 -> Scope3/1, Product11/1
  l_r1/1 -> Product9/2
  From1/1 -> Divide2/1
  Product8/1 -> Add9/1
  From2/1 -> Square/1
  l_f1/1 -> Product8/1
  Constant4/1 -> Gain3/1, Product5/2
  Product3/1 -> Divide1/1
  Divide1/1 -> Add7/1
  Wheelbase/1 -> Product4/1
  Constant/1 -> Product8/2, Product9/1
  Add7/1 -> Divide2/2
  mass/1 -> Product7/1
  [DesYawRtVal] -> Scope/1
  Product9/1 -> Add9/2
  From11/1 -> Product11/2
  [YawRtVal] -> Scope/2
  From31/1 -> To Workspace/1
  From32/1 -> To Workspace1/1
  From34/1 -> To Workspace2/1
  From33/1 -> To Workspace3/1
  Constant1/1 -> Divide/2
  [CorrYawMmtVal] -> Gain5/1, Gain6/1
  Gain6/1 -> Divide3/1
  Gain5/1 -> Divide/1
  Constant2/1 -> Divide3/2
  [state] -> Compare To Constant/1
  [CorrYawCtrlRearTq] -> Saturation4/1
  [YawCtrlRearTq] -> Delay2/1
  [YawCtrlFrntTq] -> Delay1/1
  Add1/1 -> Mux3/1
  Add2/1 -> Mux3/2
  Delay1/1 -> Add1/1
  [CorrYawCtrlFrntTq] -> Saturation1/1
  Mux3/1 -> Product/1
  Delay2/1 -> Add2/1
  Compare To Constant/1 -> Product/2
  [state] -> Compare To Constant1/1
  [CorrYawCtrlRearTq] -> Saturation5/1
  [YawCtrlRearTq] -> Delay8/1
  [MotTqCmdFrntVal] -> Delay3/1
  Delay3/1 -> Mux4/1
  Add4/1 -> Mux4/2
  Delay8/1 -> Add4/1
  [OvrStrFlag] -> Switch1/2
  Mux4/1 -> Switch1/1
  Switch1/1 -> Product1/1
  Mux5/1 -> Switch1/3
  [YawCtrlRearTq] -> Delay10/1
  Delay10/1 -> Add5/1
  [CorrYawCtrlRearTq] -> Gain4/1
  Add5/1 -> Mux5/2
  [MotTqCmdFrntVal] -> Delay9/1
  Delay9/1 -> Mux5/1
  Compare To Constant1/1 -> Product1/2
  [MotTqCmdRearVal] -> Delay13/1
  [YawCtrlFrntTq] -> Delay6/1
  [state] -> Compare To Constant2/1
  Compare To Constant2/1 -> Product2/2
  Switch3/1 -> Product2/1
  Mux6/1 -> Switch3/1
  [OvrStrFlag] -> Switch3/2
  Mux7/1 -> Switch3/3
  [CorrYawCtrlFrntTq] -> Gain/1
  Add3/1 -> Mux6/1
  Delay13/1 -> Mux6/2
  [CorrYawCtrlFrntTq] -> Saturation8/1
  Add8/1 -> Mux7/1
  [MotTqCmdRearVal] -> Delay14/1
  [YawCtrlFrntTq] -> Delay11/1
  Delay14/1 -> Mux7/2
  Delay11/1 -> Add8/2
  Gain/1 -> Saturation7/1
  Product/1 -> Scope6/1, Add/1
  Product1/1 -> Add/2
  Product2/1 -> Scope4/1, Add/3
  [CorrYawMmtVal] -> Relational Operator/1
  Constant3/1 -> Relational Operator/2
  Relational Operator/1 -> [OvrStrFlag]
  From22/1 -> To Workspace4/1
  [YawRtVal] -> Sum2/2
  [DesYawRtVal] -> Sum2/1
  Sum2/1 -> Scope1/1, Discrete Transfer Fcn/1, DiscreteIntegrator_ExtRst2/1(U), Gain2/1
  Discrete Transfer Fcn/1 -> Sum/3
  DiscreteIntegrator_ExtRst2/1(Y) -> Sum/2
  Gain2/1 -> Sum/1
  Sum/1 -> [CorrYawMmtVal], PID Control1/1
  [DesYawRtVal] -> DesYawRtVal/1
  [YawCtrlFrntTq_] -> YawCtrlFrntTq/1
  [YawCtrlRearTq_] -> YawCtrlRearTq/1
  [CorrYawMmtVal] -> CorrYawMmtVal/1
  YawRtVal/1 -> [YawRtVal]
  MotTqCmdFrntVal/1 -> [MotTqCmdFrntVal]
  MotTqCmdRearVal/1 -> [MotTqCmdRearVal]
  State/1 -> [state]
  Gain4/1 -> Saturation6/1
  Product11/1 -> Goto/1
  Des_YawRtVal/1 -> [DesYawRtVal]
  RegenCmdTq/1 -> [RegenCmdTq]
  Divide/1 -> [CorrYawCtrlFrntTq], Scope2/1
  Divide3/1 -> [CorrYawCtrlRearTq], Scope2/2
  Saturation1/1 -> Add1/2
  Saturation4/1 -> Add2/2
  Saturation5/1 -> Add4/2
  Saturation6/1 -> Add5/2
  Saturation7/1 -> Add3/1
  Saturation8/1 -> Add8/1
  [YawCtrlRearTq] -> Add10/2
  [YawCtrlFrntTq] -> Add10/1
  Add10/1 -> Relational Operator1/1
  [RegenCmdTq] -> Relational Operator1/2
  Relational Operator1/1 -> Switch/2
  Switch/1 -> Demux/1
  [MotTqCmdRearVal] -> Delay5/1
  Delay5/1 -> Mux/2
  [MotTqCmdFrntVal] -> Delay4/1
  Delay4/1 -> Mux/1
  Mux/1 -> Switch/1
  [YawCtrlFrntTq] -> Mux1/1
  [YawCtrlRearTq] -> Mux1/2
  Mux1/1 -> Switch/3
  Demux/1 -> [YawCtrlFrntTq_]
  Demux/2 -> [YawCtrlRearTq_]
  [YawCtrlFrntTq_] -> Mux8/1
  [YawCtrlRearTq_] -> Mux8/2
  Mux8/1 -> Scope5/1
  Yaw Flag/1 -> [YawFlag]
  Demux1/1 -> Rate Limiter/1(In)
  Switch2/1 -> Demux1/1
  Saturation3/1 -> [YawCtrlRearTq]
  Rate Limiter/1(Out) -> Saturation2/1
  Saturation2/1 -> [YawCtrlFrntTq]
  Demux1/2 -> Rate Limiter1/1(In)
  Rate Limiter1/1(Out) -> Saturation3/1
  [YawFlag] -> Switch2/2
  Add/1 -> Switch2/1
  [MotTqCmdRearVal] -> Delay12/1
  Mux2/1 -> Switch2/3
  Delay6/1 -> Add3/2
  [MotTqCmdFrntVal] -> Delay7/1
  Delay7/1 -> Mux2/1
  Delay12/1 -> Mux2/2

== system S250205simul_switch_2023a/Regen, Tb_max1/Triggered Subsystem2 ==
  In1 : Inport
  Trigger : TriggerPort  VariantControl=(inherit)
  Out1 : Outport
  wires:
  In1/1 -> Out1/1

== system S250205simul_switch_2023a/Regen, Tb_max1/Triggered Subsystem3 ==
  In1 : Inport
  Trigger : TriggerPort  VariantControl=(inherit)
  Out1 : Outport
  wires:
  In1/1 -> Out1/1

== system S250205simul_switch_2023a/Regen, Tb_max1/Triggered Subsystem6 ==
  In1 : Inport
  Trigger : TriggerPort  VariantControl=(inherit)
  Out1 : Outport
  wires:
  In1/1 -> Out1/1

== system S250205simul_switch_2023a/Regen, Tb_max1/Triggered Subsystem9 ==
  In1 : Inport
  Trigger : TriggerPort  VariantControl=(inherit)
  Out1 : Outport
  wires:
  In1/1 -> Out1/1

== system S250205simul_switch_2023a/Slip Control State1/Subsystem ==
  Phs_L : Inport
  Tq_L : Inport  Port=2
  Phs_R : Inport  Port=3
  Tq_R : Inport  Port=4
  Max : MinMax  Function=max  Inputs=2
  Switch : Switch  Criteria=u2 > Threshold  Threshold=1  SaturateOnIntegerOverflow=off  InputSameDT=off
  Switch1 : Switch  Criteria=u2 > Threshold  Threshold=1  SaturateOnIntegerOverflow=off  InputSameDT=off
  Tq : Outport
  wires:
  Phs_L/1 -> [Phs_L]
  Tq_L/1 -> [Tq_L]
  Phs_R/1 -> [Phs_R]
  Tq_R/1 -> [Tq_R]
  [Phs_L] -> Switch/2
  [Tq_L] -> Switch/1
  [Tq_R] -> Switch/3
  [Tq_L] -> Switch1/3
  [Tq_R] -> Switch1/1
  [Phs_R] -> Switch1/2
  Switch/1 -> Max/1
  Switch1/1 -> Max/2
  Max/1 -> Tq/1

== system S250205simul_switch_2023a/Slip Control State1/Subsystem1 ==
  Phs_L : Inport
  Tq_L : Inport  Port=2
  Phs_R : Inport  Port=3
  Tq_R : Inport  Port=4
  Max : MinMax  Function=max  Inputs=2
  Switch : Switch  Criteria=u2 > Threshold  Threshold=1  SaturateOnIntegerOverflow=off  InputSameDT=off
  Switch1 : Switch  Criteria=u2 > Threshold  Threshold=1  SaturateOnIntegerOverflow=off  InputSameDT=off
  Tq : Outport
  wires:
  Phs_L/1 -> [Phs_L]
  Tq_L/1 -> [Tq_L]
  Phs_R/1 -> [Phs_R]
  Tq_R/1 -> [Tq_R]
  [Phs_L] -> Switch/2
  [Tq_L] -> Switch/1
  [Tq_R] -> Switch/3
  [Tq_L] -> Switch1/3
  [Tq_R] -> Switch1/1
  [Phs_R] -> Switch1/2
  Switch/1 -> Max/1
  Switch1/1 -> Max/2
  Max/1 -> Tq/1
